simulink model "das2xpctest"  (Simulink 6.6)
settings: Solver=ode4  StartTime=0.0  StopTime=30  FixedStep=Auto  RelTol=1e-3
libraries: xpclib x5
settings Model: Creator=chadwick  LastModifiedBy=admin  SimulationMode=external  ParamWorkspaceSource=ReferencedWorkspace  ExtModeAutoUpdateStatusClock=off  BufferReuse=off  ProdHWDeviceType=32-bit xPC Target (Intel Pentium)
settings DataIOCC: MaxDataPoints=20000  SaveOutput=off  SignalLogging=off  SaveTime=off
settings OptimizationCC: BlockReduction=off  InlineParams=on  OptimizeBlockIOStorage=off  BufferReuse=off  ExpressionFolding=off  LocalBlockOutputs=off
settings DebuggingCC: SignalResolutionControl=TryResolveAllWithWarning  MultiTaskDSMMsg=warning  MultiTaskCondExecSysMsg=none
settings HardwareCC: ProdIntDivRoundTo=Zero  ProdEndianess=LittleEndian  ProdHWDeviceType=32-bit xPC Target (Intel Pentium)
settings ModelReferenceCC: ModelReferenceNumInstancesAllowed=Single
settings RTWCC: SystemTargetFile=xpctarget.tlc  TemplateMakefile=xpc_default_tmf  Description=xPC Target  ProcessScript=xpctarget_make_rtw_hook  CustomInclude=..\..\sdbio\ ..\model\  CustomSource=sdbio.c sdlib.c model_d.c  IncludeERTFirstTime=on
settings xpcTargetCC: TargetFcnLib=ansi_tfl_tmw.mat  GenFloatMathFcnCalls=ANSI_C  PortableWordSizes=off  RL32LogBufSizeModifier=20000

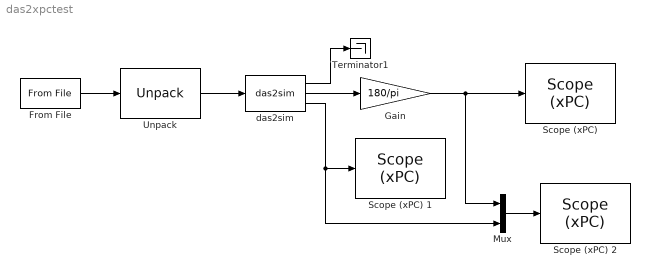
== system das2xpctest ==
  From File : xpclib/Misc./From File  filename='infile'  dataSize=816  bufSize=40000  readSize=4096  EOFOption=Hold last output  sampTime=0.001
  Gain : Gain  Gain=180/pi
  Mux : Mux  Inputs=2
  "Scope (xPC) " : xpclib/Misc./Scope (xPC)   SystemSampleTime=-1  scopeno=1  scopetype=Target  autostart=on  viewmode=Graphical rolling  formatstr='%15.6f'  grid=on  ylimits=[0,0]  nosamples=300  noprepostsamples=0  interleave=10  triggermode=FreeRun  triggersignal=1  triggerlevel=0.0  triggerslope=Either  triggerscope=1  triggersample=0  filename=angles.dat  mode=Lazy  writesize=512  autorestart=off
  Scope (xPC) 1 : xpclib/Misc./Scope (xPC)   SystemSampleTime=-1  scopeno=2  scopetype=Target  autostart=on  viewmode=Graphical rolling  formatstr='%15.6f'  grid=on  ylimits=[0,1]  nosamples=300  noprepostsamples=0  interleave=10  triggermode=FreeRun  triggersignal=1  triggerlevel=0.0  triggerslope=Either  triggerscope=1  triggersample=0  filename=ghstab.dat  mode=Lazy  writesize=512  autorestart=off
  Scope (xPC) 2 : xpclib/Misc./Scope (xPC)   SystemSampleTime=-1  scopeno=3  scopetype=File  autostart=on  viewmode=Graphical rolling  formatstr='%15.6f'  grid=on  ylimits=[0,1]  nosamples=3000  noprepostsamples=0  interleave=10  triggermode=FreeRun  triggersignal=1  triggerlevel=0.0  triggerslope=Either  triggerscope=1  triggersample=0  filename=data.dat  mode=Lazy  writesize=512  autorestart=off
  Terminator1 : Terminator
  Unpack : xpclib/UDP/Unpack  dimensions={[102]}  datatypes={'double'}  byteAlign=1
  das2sim : S-Function  FunctionName=das2sim
  wires:
  das2sim/1 -> Terminator1/1
  das2sim/2 -> Gain/1
  Gain/1 -> "Scope (xPC) "/1, Mux/1
  das2sim/3 -> Scope (xPC) 1/1, Mux/2
  From File/1 -> Unpack/1
  Unpack/1 -> das2sim/1
  Mux/1 -> Scope (xPC) 2/1
